simulink model "simulinkRobust"  (R2020b)
settings: Solver=VariableStepAuto  StartTime=0.0  StopTime=20  RelTol=1e-3
libraries: simulink_extras x5, cstblocks x2
settings Model: Creator=piero  LastModifiedBy=piero

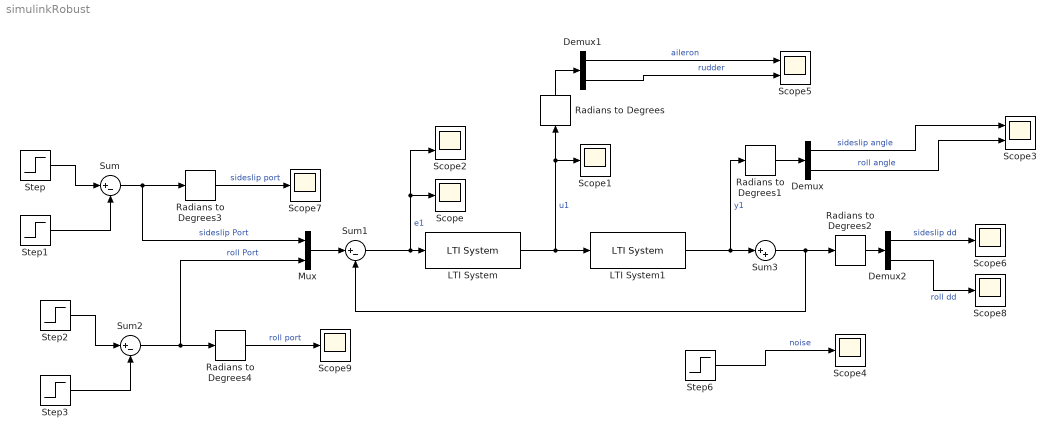
== system simulinkRobust ==
  Demux : Demux  Outputs=2
  Demux1 : Demux  Outputs=2
  Demux2 : Demux  Outputs=2
  LTI System : cstblocks/LTI System  sys=K6  IC=[]
  LTI System1 : cstblocks/LTI System  sys=P1  IC=[]
  Mux : Mux  Inputs=2
  Radians to Degrees{,1..4} (5 alike) : simulink_extras/Transformations/Radians to Degrees
  Scope{,1,4,6..9} (7 alike) : Scope
  Scope2 : Scope  NumInputPorts=2
  Scope3 : Scope  NumInputPorts=2
  Scope5 : Scope  NumInputPorts=2
  Step : Step  Time=4  After=pi/90  SampleTime=0
  Step1 : Step  Time=6  After=pi/90  SampleTime=0  ZeroCross=off
  Step2 : Step  Time=8  After=pi/27  SampleTime=0
  Step3 : Step  Time=12  After=pi/27  SampleTime=0  ZeroCross=off
  Step6 : Step  Time=2  After=0.02  SampleTime=0  ZeroCross=off
  Sum : Sum  Inputs=|+-
  Sum1 : Sum  Inputs=|+-
  Sum2 : Sum  Inputs=|+-
  Sum3 : Sum  Inputs=|++
  wires:
  LTI System/1 -> Radians to Degrees/1, Scope1/1, LTI System1/1  "u1"
  Sum1/1 -> Scope2/2, Scope/1, LTI System/1  "e1"
  LTI System1/1 -> Sum3/1, Radians to Degrees1/1  "y1"
  Step/1 -> Sum/1
  Step1/1 -> Sum/2
  Demux/1 -> Scope3/1  "sideslip angle"
  Demux/2 -> Scope3/2  "roll angle"
  Demux1/2 -> Scope5/2  "rudder"
  Mux/1 -> Sum1/1
  Sum/1 -> Radians to Degrees3/1, Mux/1  "sideslip Port"
  Step3/1 -> Sum2/2
  Step2/1 -> Sum2/1
  Sum2/1 -> Radians to Degrees4/1, Mux/2  "roll Port"
  Demux2/1 -> Scope6/1  "sideslip dd"
  Demux2/2 -> Scope8/1  "roll dd"
  Step6/1 -> Scope4/1  "noise"
  Radians to Degrees/1 -> Demux1/1
  Radians to Degrees1/1 -> Demux/1
  Radians to Degrees2/1 -> Demux2/1
  Sum3/1 -> Radians to Degrees2/1, Sum1/2
  Radians to Degrees3/1 -> Scope7/1  "sideslip port"
  Radians to Degrees4/1 -> Scope9/1  "roll port"
  Demux1/1 -> Scope5/1  "aileron"
